simulink model "Mag_Sensor_SensorProcessing_Test"  (R2018b)
settings: Solver=VariableStepAuto  StartTime=0.0  StopTime=1  RelTol=1e-3
libraries: magnetometer_lib x3, aerolibutil x2, Maggyro_Processing_mask x1
settings Model: Creator=Nick's PC  LastModifiedBy=Nick's PC

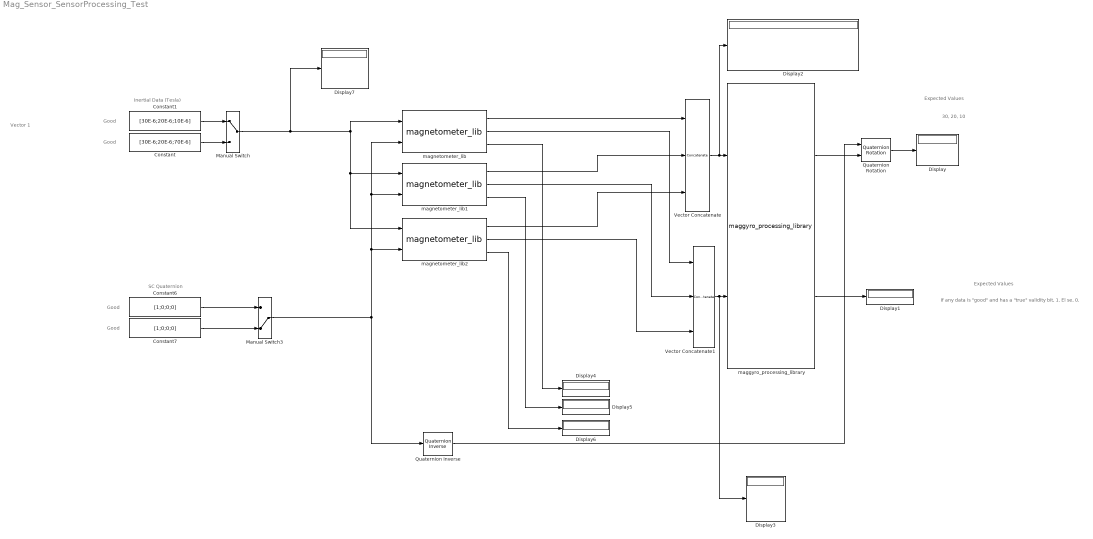
== system Mag_Sensor_SensorProcessing_Test ==
  note: Inertial Data (Tesla)
  note: Vector 1
  note: 30, 20, 10
  note: If any data is "good" and has a "true" validity bit, 1. El se, 0.
  note: Expected Values
  note: Good
  note: Good
  note: Good
  note: Good
  note: Expected Values
  note: SC Quaternion
  Constant : Constant  Value=[30E-6;20E-6;70E-6]
  Constant1 : Constant  Value=[30E-6;20E-6;10E-6]
  Constant6 : Constant  Value=[1;0;0;0]
  Constant7 : Constant  Value=[1;0;0;0]
  Display{,1..7} (8 alike) : Display
  Manual Switch : ManualSwitch
  Manual Switch3 : ManualSwitch  CurrentSetting=0
  Quaternion Inverse : aerolibutil/Quaternion Inverse
      settings: SourceProductName=Aerospace Blockset
  Quaternion Rotation : aerolibutil/Quaternion Rotation
  Vector Concatenate : Concatenate  NumInputs=3  Mode=Multidimensional array  ConcatenateDimension=2
  Vector Concatenate1 : Concatenate  NumInputs=3  ConcatenateDimension=2
  maggyro_processing_library : Maggyro_Processing_mask/maggyro_processing_library  static_range_max_value=fswParams.sensors.mag_static_range  offset_calibration_matrix=fswParams.sensors.mag_offset  mag_max_err=fswParams.sensors.mag_max_err  rotation_calibration_matrix=fswParams.sensors.mag_rotate
      link override Data Calibration/Variable Selector1: Elements=[2]
      link override Data Calibration/Variable Selector2: Elements=[3]
  magnetometer_lib : magnetometer_lib/magnetometer_lib  id_s=1  rotation_calibration_matrix=fswParams.sensors.mag_rotate  offset_calibration_matrix=fswParams.sensors.mag_offset
  magnetometer_lib1 : magnetometer_lib/magnetometer_lib  id_s=2  rotation_calibration_matrix=fswParams.sensors.mag_rotate  offset_calibration_matrix=fswParams.sensors.mag_offset
  magnetometer_lib2 : magnetometer_lib/magnetometer_lib  id_s=3  rotation_calibration_matrix=fswParams.sensors.mag_rotate  offset_calibration_matrix=fswParams.sensors.mag_offset
  wires:
  maggyro_processing_library/2 -> Display1/1
  Constant1/1 -> Manual Switch/1
  Constant/1 -> Manual Switch/2
  Constant6/1 -> Manual Switch3/1
  Constant7/1 -> Manual Switch3/2
  maggyro_processing_library/1 -> Quaternion Rotation/2
  Quaternion Rotation/1 -> Display/1
  Quaternion Inverse/1 -> Quaternion Rotation/1
  Manual Switch/1 -> Display7/1, magnetometer_lib/1, magnetometer_lib2/1, magnetometer_lib1/1
  Manual Switch3/1 -> Quaternion Inverse/1, magnetometer_lib2/2, magnetometer_lib1/2, magnetometer_lib/2
  magnetometer_lib/1 -> Vector Concatenate/1
  magnetometer_lib1/1 -> Vector Concatenate/2
  magnetometer_lib2/1 -> Vector Concatenate/3
  Vector Concatenate/1 -> Display2/1, maggyro_processing_library/1
  magnetometer_lib2/3 -> Display6/1
  magnetometer_lib1/3 -> Display5/1
  magnetometer_lib/3 -> Display4/1
  Vector Concatenate1/1 -> Display3/1, maggyro_processing_library/2
  magnetometer_lib2/2 -> Vector Concatenate1/3
  magnetometer_lib1/2 -> Vector Concatenate1/2
  magnetometer_lib/2 -> Vector Concatenate1/1
